simulink model "Task1"  (R2019b)
settings: Solver=VariableStepAuto  StartTime=0.0  StopTime=10.0  RelTol=1e-3
libraries: dspsrcs4 x1
settings Model: Creator=matvey  LastModifiedBy=matvey

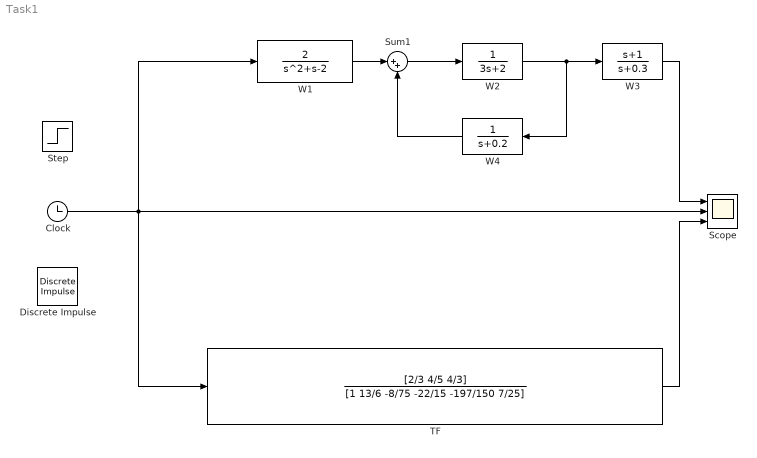
== system Task1 ==
  Clock : Clock
  Discrete Impulse : dspsrcs4/Discrete  Impulse  Delay=0  SampleTime=1  FrameSample=1  OutputFrames=off  dataType=double  isSigned=on  wordLen=16  udDataType=sfix(16)  fracBitsMode=Best precision  numFracBits=15  OutDataTypeStr=double  LastOutDataTypeStr=double
  Scope : Scope  NumInputPorts=3
  Step : Step  SampleTime=0
  Sum1 : Sum  Inputs=|++
  TF : TransferFcn  Numerator=[2/3 4/5 4/3]  Denominator=[1 13/6 -8/75 -22/15 -197/150 7/25]
  W1 : TransferFcn  Numerator=[2]  Denominator=[1 1 -2]
  W2 : TransferFcn  Denominator=[3 2]
  W3 : TransferFcn  Numerator=[1 1]  Denominator=[1 0.3]
  W4 : TransferFcn  Denominator=[1 0.2]
  wires:
  W3/1 -> Scope/1
  W1/1 -> Sum1/1
  TF/1 -> Scope/3
  W2/1 -> W4/1, W3/1
  Sum1/1 -> W2/1
  Clock/1 -> TF/1, Scope/2, W1/1
  W4/1 -> Sum1/2
